simulink model "closedLoopModel"  (R2018a)
settings: Solver=VariableStepAuto  StartTime=0.0  StopTime=100  RelTol=1e-3
libraries: simulink x1
settings Model: Creator=diogo  LastModifiedBy=diogo

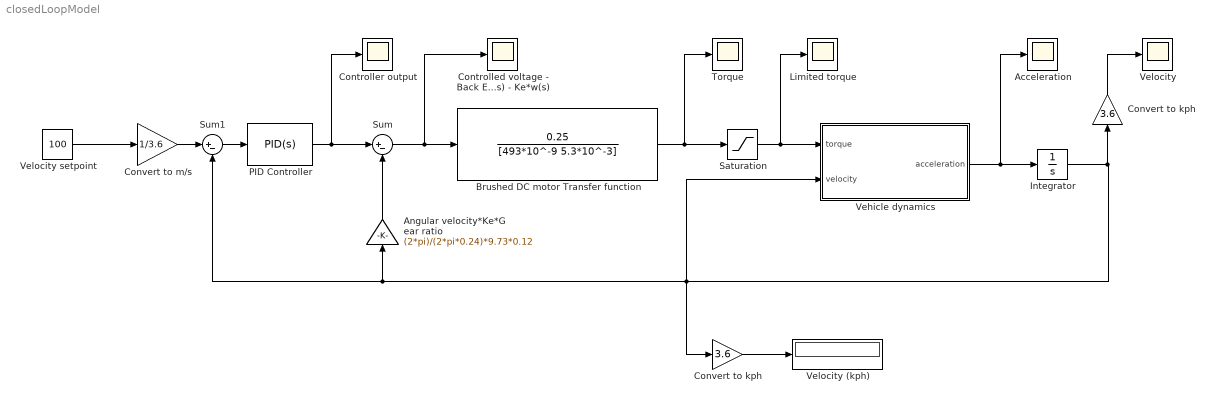
== system closedLoopModel ==
  Acceleration : Scope
  Angular velocity*Ke*Gear ratio : Gain  Gain=(2*pi)/(2*pi*0.24)*9.73*0.12
  Brushed DC motor Transfer function : TransferFcn  Numerator=[0.25]  Denominator=[493*10^-9 5.3*10^-3]
  Controlled voltage - Back EMF V(s) - Ke*w(s) : Scope
  Controller output : Scope
  Convert to kph : Gain  Gain=3.6
  "Convert to kph " : Gain  Gain=3.6
  Convert to m/s : Gain  Gain=1/3.6
  "Integrator " : Integrator
  Limited torque : Scope
  "PID Controller " : simulink/Continuous/PID Controller  Controller=PID  TimeDomain=Continuous-time  SampleTime=-1  IntegratorMethod=Forward Euler  FilterMethod=Forward Euler  Form=Parallel  UseFilter=on  ControllerParametersSource=internal  P=1000  I=200  D=1000  N=100  InitialConditionSource=internal  InitialConditionForIntegrator=0  InitialConditionForFilter=0  ExternalReset=none  LimitOutput=on  UpperSaturationLimit=346  LowerSaturationLimit=0  LinearizeAsGain=on  AntiWindupMode=clamping  Kb=1  TrackingMode=off  Kt=1  PParamMin=[]  PParamMax=[]  IParamMin=[]  IParamMax=[]  DParamMin=[]  DParamMax=[]  NParamMin=[]  NParamMax=[]  KbParamMin=[]  KbParamMax=[]  KtParamMin=[]  KtParamMax=[]  POutMin=[]  POutMax=[]  IOutMin=[]  IOutMax=[]  DOutMin=[]  DOutMax=[]  NOutMin=[]  NOutMax=[]  KbOutMin=[]  KbOutMax=[]  KtOutMin=[]  KtOutMax=[]  IntegratorOutMin=[]  IntegratorOutMax=[]  FilterOutMin=[]  FilterOutMax=[]  SumOutMin=[]  SumOutMax=[]  SumI1OutMin=[]  SumI1OutMax=[]  SumI2OutMin=[]  SumI2OutMax=[]  SumI3OutMin=[]  SumI3OutMax=[]  SumDOutMin=[]  SumDOutMax=[]  SaturationOutMin=[]  SaturationOutMax=[]  IntegratorContinuousStateAttributes=''  IntegratorStateMustResolveToSignalObject=off  IntegratorRTWStateStorageClass=Auto  FilterContinuousStateAttributes=''  FilterStateMustResolveToSignalObject=off  FilterRTWStateStorageClass=Auto  DifferentiatorICPrevScaledInput=0  DifferentiatorOutMin=[]  DifferentiatorOutMax=[]  FilterDiffOutCoefMin=[]  FilterDiffOutCoefMax=[]  SumDenOutMin=[]  SumDenOutMax=[]  SumNumOutMin=[]  SumNumOutMax=[]  ReciprocalOutMin=[]  ReciprocalOutMax=[]  DivideOutMin=[]  DivideOutMax=[]  TunerSelectOption=Transfer Function Based (PID Tuner App)
  "Saturation " : Saturate  UpperLimit=601  LowerLimit=0
  Sum : Sum  Inputs=|+-
  Sum1 : Sum  Inputs=|+-
  Torque : Scope
  Vehicle dynamics : MATLAB Function  TreatAsAtomicUnit=on
  Velocity : Scope
  Velocity (kph) : Display
  Velocity setpoint : Constant  Value=100
  wires:
  "PID Controller "/1 -> Sum/1, Controller output/1
  Angular velocity*Ke*Gear ratio/1 -> Sum/2
  Sum/1 -> Brushed DC motor Transfer function/1, Controlled voltage - Back EMF V(s) - Ke*w(s)/1
  Brushed DC motor Transfer function/1 -> Torque/1, "Saturation "/1
  Vehicle dynamics/1(acceleration) -> Acceleration/1, "Integrator "/1
  "Integrator "/1 -> Sum1/2, Angular velocity*Ke*Gear ratio/1, Vehicle dynamics/2(velocity), Convert to kph/1, "Convert to kph "/1
  Convert to kph/1 -> Velocity (kph)/1
  "Saturation "/1 -> Vehicle dynamics/1(torque), Limited torque/1
  Convert to m/s/1 -> Sum1/1
  Sum1/1 -> "PID Controller "/1
  Velocity setpoint/1 -> Convert to m/s/1
  "Convert to kph "/1 -> Velocity/1

== matlab function closedLoopModel/Vehicle dynamics ==
  data: torque input; acceleration output; velocity input
function acceleration = fcn(torque, velocity)
acceleration = (40.5*torque*0.6 - 413 - 0.3381*velocity^2)/2108;
